simulink model "FOC_PIL_Algth_top"  (R2022b)
settings: Solver=FixedStepAuto  StartTime=0.0  StopTime=4  FixedStep=Ts_PIL  RelTol=1e-3
values from neighbouring files (symbols this model uses):
  Tctr = Ts    (= 5e-05)    [FOC_Config.m]
undefined symbols (not defined in the file or in its folder): motor
libraries: mcbplantlib x1, autolibpmsminterior x1
settings Model: Creator=k  LastModifiedBy=Administrator
settings SolverCC: AlgebraicLoopSolver=TrustRegion
settings DebuggingCC: UnconnectedInputMsg=warning  UnconnectedOutputMsg=warning  UnconnectedLineMsg=warning  SFMachineParentedDataDiag=warning
settings ModelReferenceCC: EnableRefExpFcnMdlSchedulingChecks=on
settings RTWCC: DLArmComputeVersion=19.05

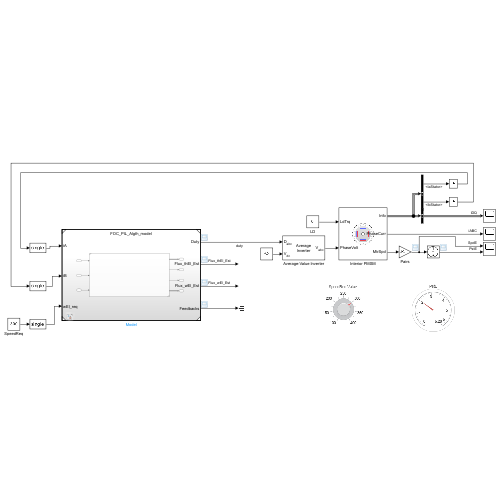
[thumbnail: Simulink's stored preview of the top-level diagram]
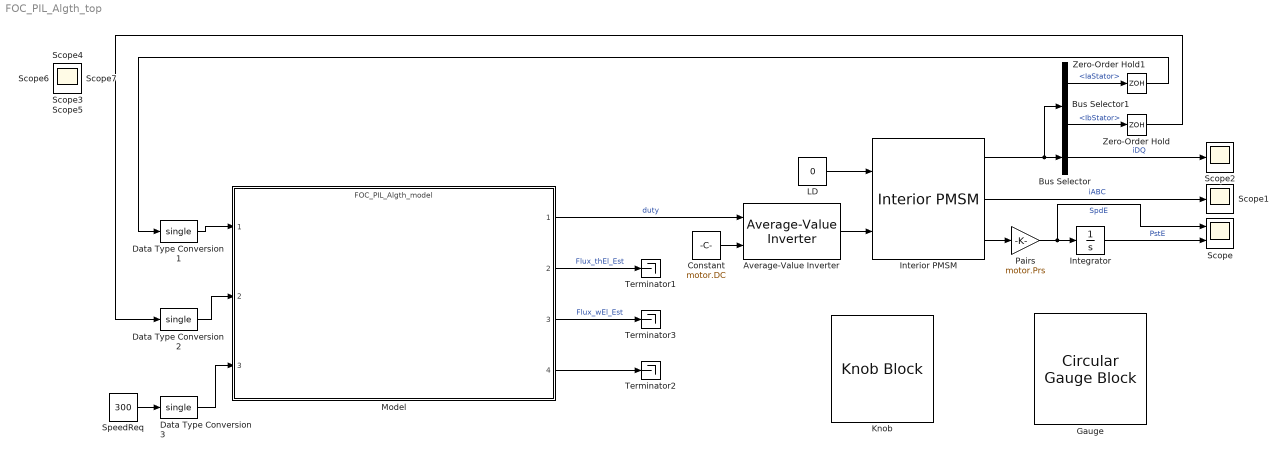
== system FOC_PIL_Algth_top ==
  Average-Value Inverter : mcbplantlib/Average-Value Inverter
  Bus Selector : BusSelector  OutputSignals=IdSync,IqSync  OutputAsBus=on
  Bus Selector1 : BusSelector  OutputSignals=IaStator,IbStator
  Constant : Constant  Value=motor.DC
  Data Type Conversion1 : DataTypeConversion  OutDataTypeStr=single  SaturateOnIntegerOverflow=off  RndMeth=Floor
  Data Type Conversion2 : DataTypeConversion  OutDataTypeStr=single  SaturateOnIntegerOverflow=off  RndMeth=Floor
  Data Type Conversion3 : DataTypeConversion  OutDataTypeStr=single  SaturateOnIntegerOverflow=off  RndMeth=Floor
  Gauge : CircularGaugeBlock  ScaleMax=6.28  TickInterval=1
  Integrator : Integrator  WrapState=on  WrappedStateUpperValue=2*pi  WrappedStateLowerValue=0
  Interior PMSM : autolibpmsminterior/Interior PMSM  port_config=Torque  sim_type=Continuous  Ts=0.001  P=motor.Prs  Rs=motor.Rs  Ldq=[motor.Ld motor.Lq]  KConstText=Permanent flux linkage constant (lambda_pm):  lambda_pm=motor.Flux  Ke=159.9771  mechanical=[motor.J, motor.B, motor.Tf]  idq0=[0 0]  theta_init=0  omega_init=0  KConst=motor.Flux  lambda_pm_calc=motor.Flux  Kt=0.07  RefBlkName='autolibpmsminterior/Interior PMSM'  aMode=5
  Knob : KnobBlock  ScaleMin=100  ScaleMax=400
  LD : Constant  Value=0
  Model : ModelReference  ModelNameDialog=FOC_PIL_Algth_model.slx  SimulationMode=Normal  ModelReferenceVersion=5.2
  Pairs : Gain  Gain=motor.Prs
  Scope : Scope  NumInputPorts=2
  Scope{1..7} (7 alike) : Scope
  SpeedReq : Constant  Value=300
  Terminator1 : Terminator
  Terminator2 : Terminator
  Terminator3 : Terminator
  Zero-Order Hold : ZeroOrderHold  SampleTime=Tctr
  Zero-Order Hold1 : ZeroOrderHold  SampleTime=Tctr
  wires:
  Bus Selector/1 -> Scope2/1  "iDQ"
  LD/1 -> Interior PMSM/1
  Interior PMSM/1 -> Bus Selector1/1, Bus Selector/1
  Bus Selector1/1 -> Zero-Order Hold1/1  "<IaStator>"
  Pairs/1 -> Integrator/1, Scope/1  "SpdE"
  Interior PMSM/2 -> Scope1/1  "iABC"
  Bus Selector1/2 -> Zero-Order Hold/1  "<IbStator>"
  Interior PMSM/3 -> Pairs/1
  Model/1 -> Average-Value Inverter/1  "duty"
  Average-Value Inverter/1 -> Interior PMSM/2
  Constant/1 -> Average-Value Inverter/2
  Data Type Conversion1/1 -> Model/1
  Data Type Conversion2/1 -> Model/2
  Data Type Conversion3/1 -> Model/3
  SpeedReq/1 -> Data Type Conversion3/1
  Model/2 -> Terminator1/1  "Flux_thEl_Est"
  Model/3 -> Terminator3/1  "Flux_wEl_Est"
  Model/4 -> Terminator2/1
  Integrator/1 -> Scope/2  "PstE"
  Zero-Order Hold/1 -> Data Type Conversion2/1
  Zero-Order Hold1/1 -> Data Type Conversion1/1
